simulink model "starshotsimv3p5"  (R2017a)
settings: Solver=ode45  StartTime=0.0  StopTime=30  MaxStep=4.0  MinStep=.001  RelTol=1e-6
values from neighbouring files (symbols this model uses):
  B0 = 3.12e-5    (= 3.12e-05)    [starshot_DC_KD_setup.m]    (also in starshot_DC_setup.m; starshotmath.m; temp.m)
  G = 6.67e-11    [starshot_DC_KD_setup.m]    (also in starshot_DC_setup.m; temp.m)
  M_Earth = 5.972e24    (= 5.972e+24)    [starshot_DC_KD_setup.m]    (also in starshot_DC_setup.m; temp.m)
  mu_0 = 4*pi*(10^-7)    (= 1.25663706144e-06)    [starshot_DC_KD_setup.m]    (also in starshot_DC_setup.m; temp.m)
  n = 1000    [starshot_DC_KD_setup.m]    (also in starshot_DC_setup.m; starshotmath.m; temp.m)
  q0 = [qmatlab(2:4),qmatlab(1)]'    [starshot_DC_KD_setup.m]    (also in starshot_DC_setup.m; temp.m)
  R_Earth = 6.378e6    (= 6378000)    [starshot_DC_KD_setup.m]    (also in starshot_DC_setup.m; temp.m)
undefined symbols (not defined in the file or in its folder): Kp_phi, omegacmd, quatcmd, starshot
libraries: vrlib x2
settings Model: Creator=armen  LastModifiedBy=armen

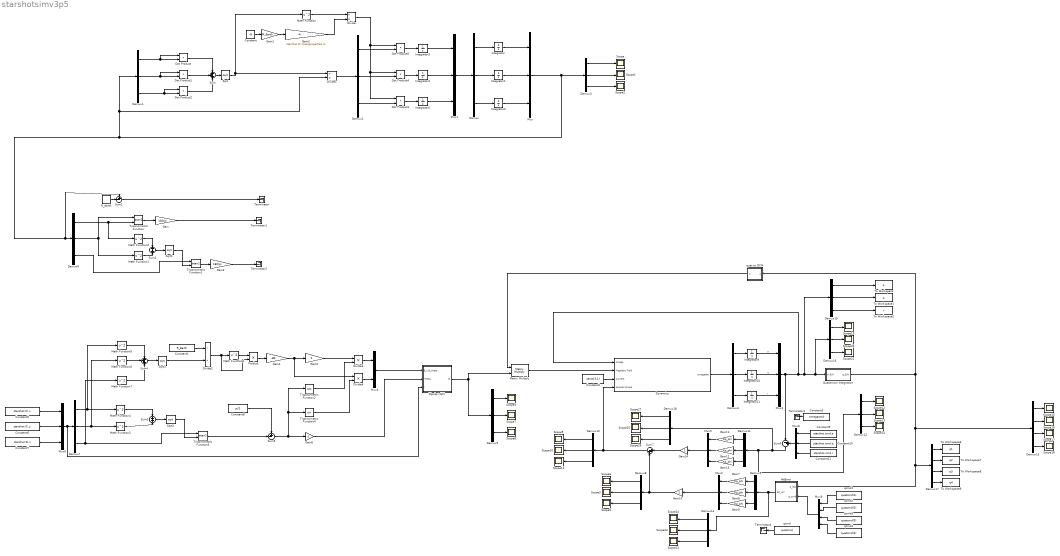
== system starshotsimv3p5 ==
  AttError : Subsystem
  Constant : Constant  Value=-G
  Constant1 : Constant  Value=R_Earth
  Constant10 : Constant  Value=starshot.cmd.q
  Constant11 : Constant  Value=starshot.cmd.r
  Constant2 : Constant  Value=zeros(3,1)
  Constant3 : Constant  Value=omegacmd
  Constant5 : Constant  Value=starshot.IC.x
  Constant6 : Constant  Value=starshot.IC.y
  Constant7 : Constant  Value=starshot.IC.z
  Constant8 : Constant  Value=pi/2
  Constant9 : Constant  Value=starshot.cmd.p
  Demux{,1..12,14..16,18} (17 alike) : Demux  Outputs=3
  Demux13 : Demux
  Demux17 : Demux
  Dipole->ECI : Subsystem
  Divide : Product  Inputs=/*
  Divide1 : Product  Inputs=/*
  Divide2 : Product  Inputs=*/
  Divide3 : Product  Inputs=**
  Divide4 : Product  Inputs=**
  Dot Product{,1..5} (6 alike) : DotProduct  InputSameDT=on  OutDataTypeStr=Inherit: Inherit via internal rule
  Dynamics : Subsystem
  Gain : Gain  Gain=180/pi
  Gain1 : Gain  Gain=M_Earth
  Gain10 : Gain
  Gain{7..9,11..13} (6 alike) : Gain  Gain=Kp_phi
  Gain14 : Gain
  Gain2 : Gain  Gain=starshot.IC.massproperties.m
  Gain3 : Gain  Gain=180/pi
  Gain4 : Gain  Gain=-B0
  Gain5 : Gain  Gain=2
  Gain6 : Gain  Gain=-1
  Integrator : Integrator  InitialCondition=starshot.IC.x
  Integrator1 : Integrator  InitialCondition=starshot.IC.y
  Integrator10 : Integrator  InitialCondition=starshot.IC.q
  Integrator11 : Integrator  InitialCondition=starshot.IC.r
  Integrator2 : Integrator  InitialCondition=starshot.IC.z
  Integrator3 : Integrator  InitialCondition=starshot.IC.xdot
  Integrator4 : Integrator  InitialCondition=starshot.IC.ydot
  Integrator5 : Integrator  InitialCondition=starshot.IC.zdot
  Integrator9 : Integrator  InitialCondition=starshot.IC.p
  Math Function{,1..8} (9 alike) : Math  Operator=square  SaturateOnIntegerOverflow=on
  Matrix Multiply : Product  Multiplication=Matrix(*)
  Mux{,1..3,5..6,8} (7 alike) : Mux  Inputs=3
  Mux4 : Mux  Inputs=2
  Mux9 : Mux
  Product : Product
  Quaternion Integration : Subsystem
  R_earth : Constant  Value=6.371e6
  Scope{,1..27} (28 alike) : Scope
  Sqrt{,1..3} (4 alike) : Sqrt  SaturateOnIntegerOverflow=on
  Sum : Sum  Inputs=+++
  Sum1 : Sum  Inputs=+-|
  Sum2 : Sum
  Sum3 : Sum
  Sum4 : Sum  Inputs=+++
  Sum5 : Sum  Inputs=+-|
  Sum6 : Sum  Inputs=|-+
  Sum7 : Sum  Inputs=|++
  Terminator{,1..4} (5 alike) : Terminator
  To Workspace : ToWorkspace  VariableName=p  SaveFormat=Timeseries  SampleTime=-1
  To Workspace1 : ToWorkspace  VariableName=q  SaveFormat=Timeseries  SampleTime=-1
  To Workspace2 : ToWorkspace  VariableName=r  SaveFormat=Timeseries  SampleTime=-1
  To Workspace6 : ToWorkspace  VariableName=q1  SaveFormat=Timeseries  SampleTime=-1
  To Workspace7 : ToWorkspace  VariableName=q2  SaveFormat=Timeseries  SampleTime=-1
  To Workspace8 : ToWorkspace  VariableName=q3  SaveFormat=Timeseries  SampleTime=-1
  To Workspace9 : ToWorkspace  VariableName=q4  SaveFormat=Timeseries  SampleTime=-1
  Trigonometric Function : Trigonometry  Operator=atan2
  Trigonometric Function1 : Trigonometry  Operator=atan2
  Trigonometric Function2 : Trigonometry  Operator=cos
  Trigonometric Function3 : Trigonometry  Operator=atan2
  Trigonometric Function4 : Trigonometry
  qcmd : Constant  Value=quatcmd
  qcmd1 : Constant  Value=quatcmd(1)
  qcmd2 : Constant  Value=quatcmd(2)
  qcmd3 : Constant  Value=quatcmd(3)
  qcmd4 : Constant  Value=quatcmd(4)
  quat to DCM : Subsystem  mask(Direction Cosine Matrix){}
      mask help: Determines the 3x3 Direction Cosine Matrix (DCM) from a 4x1 quaternion orientation vector. The outputted DCM transforms vectors from inertial axes to body axes. This version corrects the fucked-up MATLAB one.
      mask Help:
      | <p>This block determines the 3x3 Direction Cosine Matrix (DCM) from a 4x1 quaternion orientation vector. The outputted DCM transforms vectors from inertial axes to body axes.  This version corrects the fucked-up MATLAB one</p>
      | 
      | <p>The block input and output contain more than one signal as described below.</p>
      | 
      | <p><H4>Block Vector Input - Quaternion</H4>
      | <ul>
      | <li>q0</li>
      | <li>q1</li>
      | <li>q2</li>
      | <li>q3</li>
      | </ul>
      | </p>
      | 
      | <p><H4>Block Matrix Output - Direction Cosine Matrix  </H4>
      |     <ul>
      |    </ul>
      |    </p>
      mask Display: disp('q to Q')
  wires:
  Integrator/1 -> Mux/1
  Integrator2/1 -> Mux/3
  Integrator1/1 -> Mux/2
  Demux/3 -> Integrator2/1
  Demux/2 -> Integrator1/1
  Demux/1 -> Integrator/1
  Mux1/1 -> Demux/1
  Integrator5/1 -> Mux1/3
  Integrator4/1 -> Mux1/2
  Integrator3/1 -> Mux1/1
  Demux1/1 -> Dot Product/1, Dot Product/2
  Demux1/2 -> Dot Product1/1, Dot Product1/2
  Demux1/3 -> Dot Product2/1, Dot Product2/2
  Dot Product1/1 -> Sum/2
  Dot Product2/1 -> Sum/3
  Dot Product/1 -> Sum/1
  Sum/1 -> Sqrt/1
  Constant/1 -> Gain1/1
  Sqrt/1 -> Math Function/1, Divide1/1
  Gain1/1 -> Gain2/1
  Gain2/1 -> Divide/2
  Math Function/1 -> Divide/1
  Divide/1 -> Dot Product3/1, Dot Product4/1, Dot Product5/1
  Demux2/3 -> Dot Product3/2
  Demux2/2 -> Dot Product4/2
  Demux2/1 -> Dot Product5/2
  Dot Product5/1 -> Integrator3/1
  Dot Product4/1 -> Integrator4/1
  Dot Product3/1 -> Integrator5/1
  Divide1/1 -> Demux2/1
  Demux3/1 -> Scope/1
  Demux3/2 -> Scope1/1
  Demux3/3 -> Scope2/1
  Integrator9/1 -> Mux3/1  "p"
  Integrator10/1 -> Mux3/2  "q"
  Integrator11/1 -> Mux3/3  "r"
  Demux4/3 -> Integrator11/1
  Demux4/2 -> Integrator10/1
  Demux4/1 -> Integrator9/1
  Sum1/1 -> Terminator/1
  R_earth/1 -> Sum1/2
  Demux6/1 -> Math Function2/1, Trigonometric Function/2
  Demux6/2 -> Trigonometric Function/1, Math Function1/1
  Demux6/3 -> Trigonometric Function1/1
  Math Function2/1 -> Sum2/1
  Math Function1/1 -> Sum2/2
  Sum2/1 -> Sqrt1/1
  Sqrt1/1 -> Trigonometric Function1/2
  Trigonometric Function/1 -> Gain/1
  Trigonometric Function1/1 -> Gain3/1
  Gain/1 -> Terminator1/1
  Gain3/1 -> Terminator2/1
  Dynamics/1(omegadot) -> Demux4/1
  Sqrt2/1 -> Trigonometric Function3/2
  Sum3/1 -> Sqrt2/1
  Math Function3/1 -> Sum3/2
  Math Function4/1 -> Sum3/1
  Demux7/3 -> Math Function7/1, Trigonometric Function3/1
  Demux7/2 -> Math Function6/1, Math Function3/1
  Demux7/1 -> Math Function5/1, Math Function4/1
  Mux/1 -> Sum1/1, Demux6/1, Divide1/2, Demux1/1, Demux3/1
  Math Function6/1 -> Sum4/2
  Math Function5/1 -> Sum4/1
  Math Function7/1 -> Sum4/3
  Sum4/1 -> Sqrt3/1
  Sqrt3/1 -> Divide2/2
  Constant1/1 -> Divide2/1
  Divide2/1 -> Product/2, Math Function8/1
  Math Function8/1 -> Product/1
  Product/1 -> Gain4/1
  Gain4/1 -> Gain5/1, Divide4/1
  Gain5/1 -> Divide3/1
  Trigonometric Function2/1 -> Divide3/2
  Trigonometric Function4/1 -> Divide4/2
  Divide3/1 -> Mux4/1
  Divide4/1 -> Mux4/2
  Mux4/1 -> Dipole->ECI/1(B_r,B_theta)
  Gain6/1 -> Dipole->ECI/2(-theta)
  Demux9/3 -> Scope8/1
  Demux9/1 -> Scope4/1
  Demux9/2 -> Scope7/1
  Dipole->ECI/1(B) -> Matrix Multiply/2, Demux9/1
  Mux6/1 -> Dipole->ECI/3(r), Demux7/1
  Constant7/1 -> Mux6/3
  Constant6/1 -> Mux6/2
  Constant5/1 -> Mux6/1
  Trigonometric Function3/1 -> Sum5/2
  Constant8/1 -> Sum5/1
  Sum5/1 -> Trigonometric Function2/1, Trigonometric Function4/1, Gain6/1
  AttError/1(att_err) -> Demux14/1, Demux5/1
  Mux2/1 -> Gain10/1
  qcmd/1 -> Terminator4/1
  Gain7/1 -> Mux2/1
  Demux5/1 -> Gain7/1
  Gain8/1 -> Mux2/2
  Demux5/2 -> Gain8/1
  Gain9/1 -> Mux2/3
  Demux5/3 -> Gain9/1
  Constant2/1 -> Dynamics/3("Current ")
  Demux10/1 -> Scope9/1
  Demux10/2 -> Scope10/1
  Demux10/3 -> Scope11/1
  Demux11/3 -> Gain13/1
  Gain13/1 -> Mux5/3
  Demux11/2 -> Gain12/1
  Gain12/1 -> Mux5/2
  Demux11/1 -> Gain11/1
  Gain11/1 -> Mux5/1
  Mux5/1 -> Gain14/1
  Constant3/1 -> Terminator3/1
  Gain14/1 -> Sum7/1
  Sum7/1 -> Dynamics/4(pseudo-torque), Demux10/1
  Demux12/3 -> Scope14/1
  Demux12/1 -> Scope12/1
  Demux12/2 -> Scope13/1
  Demux13/1 -> Scope15/1
  Demux13/4 -> Scope18/1
  Demux13/3 -> Scope17/1
  Quaternion Integration/1(q_B/N) -> Demux13/1, AttError/1(q_est), Demux17/1, quat to DCM/1(e0 e1 e2 e3)
  Demux13/2 -> Scope16/1
  Demux15/3 -> To Workspace2/1
  Demux15/2 -> To Workspace1/1
  Demux15/1 -> To Workspace/1
  Sum6/1 -> Demux18/1, Demux12/1, Demux11/1
  Demux17/3 -> To Workspace8/1
  Demux17/2 -> To Workspace7/1
  Demux17/1 -> To Workspace6/1
  Demux17/4 -> To Workspace9/1
  Mux8/1 -> Sum6/2
  Constant10/1 -> Mux8/2
  Constant11/1 -> Mux8/3
  Constant9/1 -> Mux8/1
  Mux9/1 -> AttError/2(q_cmd)
  qcmd1/1 -> Mux9/1
  qcmd2/1 -> Mux9/2
  qcmd3/1 -> Mux9/3
  qcmd4/1 -> Mux9/4
  Mux3/1 -> Demux16/1, Quaternion Integration/1(w B/N), Demux15/1, Dynamics/1(omega), Sum6/1
  Demux16/2 -> Scope20/1
  Demux16/1 -> Scope19/1
  Demux16/3 -> Scope21/1
  quat to DCM/1(DCM) -> Matrix Multiply/1
  Matrix Multiply/1 -> Dynamics/2(Magnetic Field)
  Gain10/1 -> Demux8/1, Sum7/2
  Demux8/3 -> Scope5/1
  Demux8/2 -> Scope3/1
  Demux8/1 -> Scope6/1
  Demux14/1 -> Scope24/1
  Demux14/2 -> Scope22/1
  Demux14/3 -> Scope23/1
  Demux18/3 -> Scope26/1
  Demux18/2 -> Scope25/1
  Demux18/1 -> Scope27/1

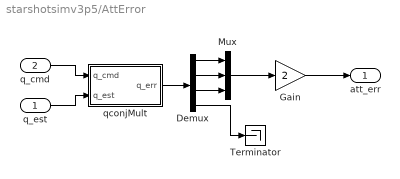
== system starshotsimv3p5/AttError ==
  q_est : Inport  PortDimensions=4
  q_cmd : Inport  Port=2  PortDimensions=4
  Demux : Demux
  Gain : Gain  Gain=2  SaturateOnIntegerOverflow=on  OutDataTypeStr=Inherit: Same as input  ParamDataTypeStr=Inherit: Same as input
  Mux : Mux  Inputs=3
  Terminator : Terminator
  qconjMult : Subsystem
  att_err : Outport
  wires:
  Demux/4 -> Terminator/1
  Gain/1 -> att_err/1
  Mux/1 -> Gain/1
  Demux/3 -> Mux/3
  Demux/2 -> Mux/2
  Demux/1 -> Mux/1
  qconjMult/1(q_err) -> Demux/1
  q_est/1 -> qconjMult/2(q_est)
  q_cmd/1 -> qconjMult/1(q_cmd)

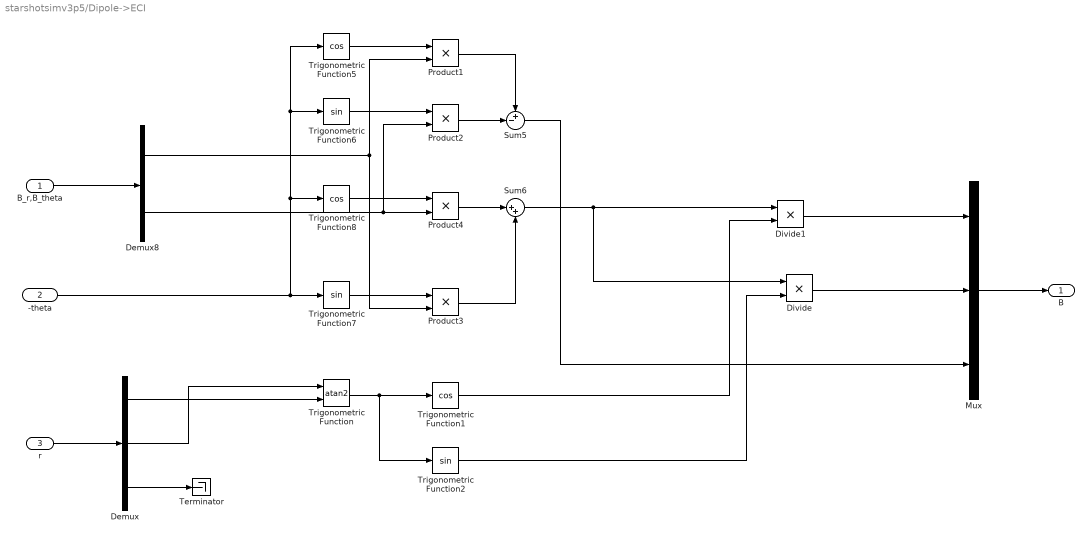
== system starshotsimv3p5/Dipole->ECI ==
  B_r,B_theta : Inport
  -theta : Inport  Port=2
  r : Inport  Port=3
  Demux : Demux  Outputs=3
  Demux8 : Demux  Outputs=2
  Divide : Product  Inputs=**
  Divide1 : Product  Inputs=**
  Mux : Mux  Inputs=3
  Product{1..4} (4 alike) : Product
  Sum5 : Sum  Inputs=+-|
  Sum6 : Sum  Inputs=|++
  Terminator : Terminator
  Trigonometric Function : Trigonometry  Operator=atan2
  Trigonometric Function1 : Trigonometry  Operator=cos
  Trigonometric Function2 : Trigonometry
  Trigonometric Function5 : Trigonometry  Operator=cos
  Trigonometric Function6 : Trigonometry
  Trigonometric Function7 : Trigonometry
  Trigonometric Function8 : Trigonometry  Operator=cos
  B : Outport
  wires:
  -theta/1 -> Trigonometric Function5/1, Trigonometric Function6/1, Trigonometric Function8/1, Trigonometric Function7/1
  Product4/1 -> Sum6/1
  Product3/1 -> Sum6/2
  Demux8/1 -> Product3/2, Product1/2
  Demux8/2 -> Product2/2, Product4/2
  Trigonometric Function5/1 -> Product1/1
  Product2/1 -> Sum5/2
  Trigonometric Function7/1 -> Product3/1
  B_r,B_theta/1 -> Demux8/1
  Sum5/1 -> Mux/3
  Trigonometric Function8/1 -> Product4/1
  Trigonometric Function6/1 -> Product2/1
  Sum6/1 -> Divide1/1, Divide/1
  Product1/1 -> Sum5/1
  r/1 -> Demux/1
  Demux/3 -> Terminator/1
  Demux/2 -> Trigonometric Function/1
  Demux/1 -> Trigonometric Function/2
  Trigonometric Function/1 -> Trigonometric Function1/1, Trigonometric Function2/1
  Trigonometric Function1/1 -> Divide1/2
  Trigonometric Function2/1 -> Divide/2
  Mux/1 -> B/1
  Divide1/1 -> Mux/1
  Divide/1 -> Mux/2

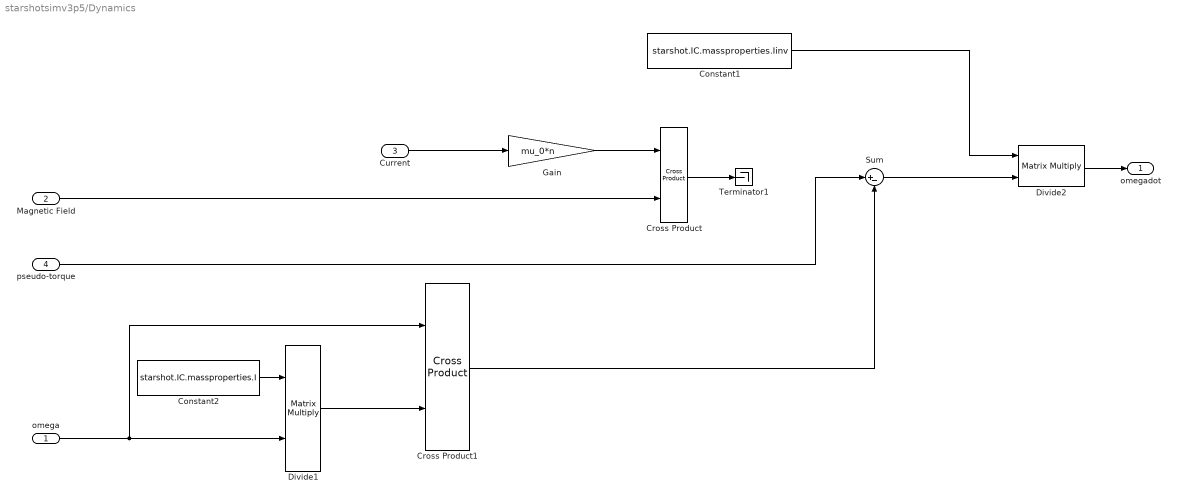
== system starshotsimv3p5/Dynamics ==
  omega : Inport
  Magnetic Field : Inport  Port=2
  "Current " : Inport  Port=3
  pseudo-torque : Inport  Port=4
  Constant1 : Constant  Value=starshot.IC.massproperties.Iinv  VectorParams1D=off
  Constant2 : Constant  Value=starshot.IC.massproperties.I  VectorParams1D=off
  Cross Product : vrlib/Utilities/Cross Product
      settings: SourceProductBaseCode=VR
  Cross Product1 : vrlib/Utilities/Cross Product
      settings: SourceProductBaseCode=VR
  Divide1 : Product  Inputs=**  Multiplication=Matrix(*)
  Divide2 : Product  Inputs=**  Multiplication=Matrix(*)
  Gain : Gain  Gain=mu_0*n
  Sum : Sum  Inputs=|+-
  Terminator1 : Terminator
  omegadot : Outport
  wires:
  omega/1 -> Divide1/2, Cross Product1/1
  Constant2/1 -> Divide1/1
  "Current "/1 -> Gain/1
  Magnetic Field/1 -> Cross Product/2
  Gain/1 -> Cross Product/1
  Cross Product/1 -> Terminator1/1
  Divide1/1 -> Cross Product1/2
  Cross Product1/1 -> Sum/2
  Sum/1 -> Divide2/2
  Constant1/1 -> Divide2/1
  Divide2/1 -> omegadot/1
  pseudo-torque/1 -> Sum/1

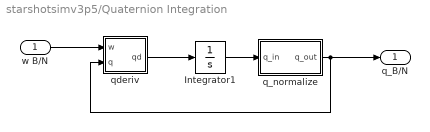
== system starshotsimv3p5/Quaternion Integration ==
  w B/N : Inport
  Integrator1 : Integrator  InitialCondition=q0
  q_normalize : Subsystem
  qderiv : Subsystem
  q_B/N : Outport
  wires:
  w B/N/1 -> qderiv/1(w)
  q_normalize/1(q_out) -> qderiv/2(q), q_B/N/1
  Integrator1/1 -> q_normalize/1(q_in)
  qderiv/1(qd) -> Integrator1/1

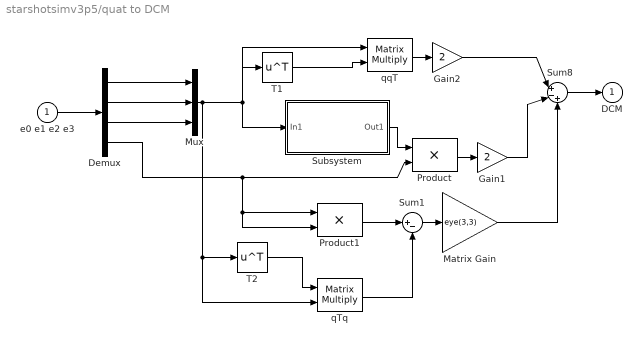
== system starshotsimv3p5/quat to DCM ==
  e0 e1 e2 e3 : Inport
  Demux : Demux
  Gain1 : Gain  Gain=2  SaturateOnIntegerOverflow=on  OutDataTypeStr=Inherit: Same as input  ParamDataTypeStr=Inherit: Same as input
  Gain2 : Gain  Gain=2  SaturateOnIntegerOverflow=on  OutDataTypeStr=Inherit: Same as input  ParamDataTypeStr=Inherit: Same as input
  Matrix Gain : Gain  Gain=eye(3,3)  SaturateOnIntegerOverflow=on  OutDataTypeStr=Inherit: Same as input  ParamDataTypeStr=Inherit: Same as input
  Mux : Mux  Inputs=3
  Product : Product  SaturateOnIntegerOverflow=on  InputSameDT=on  OutDataTypeStr=Inherit: Same as first input
  Product1 : Product  SaturateOnIntegerOverflow=on  InputSameDT=on  OutDataTypeStr=Inherit: Same as first input
  Subsystem : Subsystem
      mask Display: disp('3x3 cross matrix')
  Sum1 : Sum  Inputs=|+-  SaturateOnIntegerOverflow=on  InputSameDT=on  OutDataTypeStr=Inherit: Same as first input
  Sum8 : Sum  Inputs=|+-+  SaturateOnIntegerOverflow=on  InputSameDT=on  OutDataTypeStr=Inherit: Same as first input
  T1 : Math  Operator=transpose  SaturateOnIntegerOverflow=on
  T2 : Math  Operator=transpose  SaturateOnIntegerOverflow=on
  qTq : Product  Multiplication=Matrix(*)  SaturateOnIntegerOverflow=on  InputSameDT=on  OutDataTypeStr=Inherit: Same as first input
  qqT : Product  Multiplication=Matrix(*)  SaturateOnIntegerOverflow=on  InputSameDT=on  OutDataTypeStr=Inherit: Same as first input
  DCM : Outport  InitialOutput=0
  wires:
  Subsystem/1(Out1) -> Product/1
  Matrix Gain/1 -> Sum8/3
  Sum1/1 -> Matrix Gain/1
  qTq/1 -> Sum1/2
  T2/1 -> qTq/1
  Product1/1 -> Sum1/1
  Gain1/1 -> Sum8/2
  Gain2/1 -> Sum8/1
  qqT/1 -> Gain2/1
  T1/1 -> qqT/2
  Product/1 -> Gain1/1
  Mux/1 -> qTq/2, T2/1, Subsystem/1(In1), qqT/1, T1/1
  Demux/4 -> Product1/2, Product1/1, Product/2
  Demux/3 -> Mux/3
  Demux/2 -> Mux/2
  Demux/1 -> Mux/1
  e0 e1 e2 e3/1 -> Demux/1
  Sum8/1 -> DCM/1

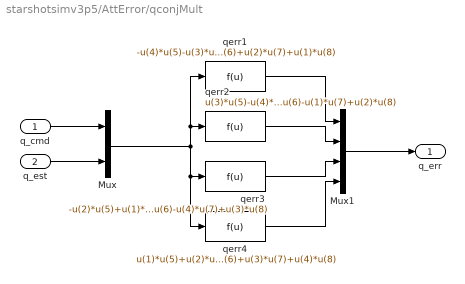
== system starshotsimv3p5/AttError/qconjMult ==
  q_cmd : Inport
  q_est : Inport  Port=2
  Mux : Mux  Inputs=2
  Mux1 : Mux
  qerr1 : Fcn  Expr=-u(4)*u(5)-u(3)*u(6)+u(2)*u(7)+u(1)*u(8)
  qerr2 : Fcn  Expr=u(3)*u(5)-u(4)*u(6)-u(1)*u(7)+u(2)*u(8)
  qerr3 : Fcn  Expr=-u(2)*u(5)+u(1)*u(6)-u(4)*u(7)+u(3)*u(8)
  qerr4 : Fcn  Expr=u(1)*u(5)+u(2)*u(6)+u(3)*u(7)+u(4)*u(8)
  q_err : Outport
  wires:
  Mux1/1 -> q_err/1
  qerr4/1 -> Mux1/4
  qerr3/1 -> Mux1/3
  qerr2/1 -> Mux1/2
  qerr1/1 -> Mux1/1
  Mux/1 -> qerr4/1, qerr3/1, qerr2/1, qerr1/1
  q_est/1 -> Mux/2
  q_cmd/1 -> Mux/1

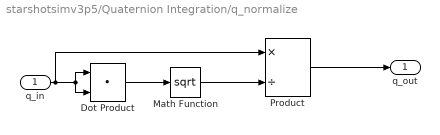
== system starshotsimv3p5/Quaternion Integration/q_normalize ==
  q_in : Inport  PortDimensions=4
  Dot Product : DotProduct  InputSameDT=on  OutDataTypeStr=Inherit: Inherit via internal rule
  Math Function : Math  Operator=sqrt  SaturateOnIntegerOverflow=on
  Product : Product  Inputs=*/  SaturateOnIntegerOverflow=on  InputSameDT=on  OutDataTypeStr=Inherit: Same as first input
  q_out : Outport
  wires:
  Product/1 -> q_out/1
  Math Function/1 -> Product/2
  Dot Product/1 -> Math Function/1
  q_in/1 -> Dot Product/2, Dot Product/1, Product/1

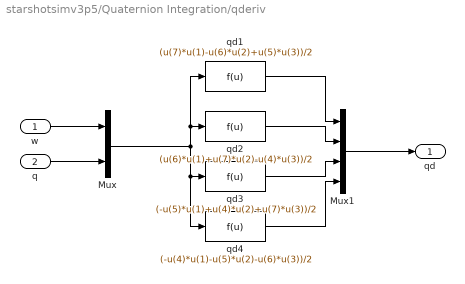
== system starshotsimv3p5/Quaternion Integration/qderiv ==
  w : Inport
  q : Inport  Port=2
  Mux : Mux  Inputs=2
  Mux1 : Mux
  qd1 : Fcn  Expr=(u(7)*u(1)-u(6)*u(2)+u(5)*u(3))/2
  qd2 : Fcn  Expr=(u(6)*u(1)+u(7)*u(2)-u(4)*u(3))/2
  qd3 : Fcn  Expr=(-u(5)*u(1)+u(4)*u(2)+u(7)*u(3))/2
  qd4 : Fcn  Expr=(-u(4)*u(1)-u(5)*u(2)-u(6)*u(3))/2
  qd : Outport
  wires:
  Mux1/1 -> qd/1
  qd4/1 -> Mux1/4
  qd3/1 -> Mux1/3
  qd2/1 -> Mux1/2
  qd1/1 -> Mux1/1
  Mux/1 -> qd4/1, qd3/1, qd2/1, qd1/1
  q/1 -> Mux/2
  w/1 -> Mux/1

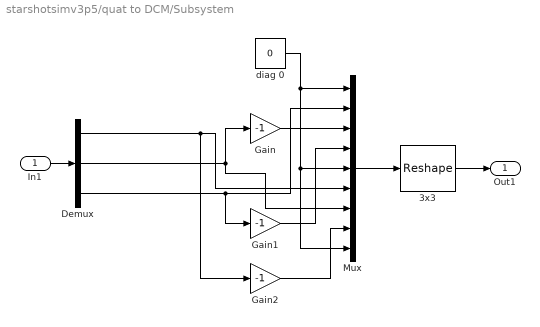
== system starshotsimv3p5/quat to DCM/Subsystem ==
  In1 : Inport
  3x3 : Reshape  OutputDimensionality=Customize  OutputDimensions=[3,3]
  Demux : Demux  Outputs=3
  Gain : Gain  Gain=-1  SaturateOnIntegerOverflow=on  OutDataTypeStr=Inherit: Same as input  ParamDataTypeStr=Inherit: Same as input
  Gain1 : Gain  Gain=-1  SaturateOnIntegerOverflow=on  OutDataTypeStr=Inherit: Same as input  ParamDataTypeStr=Inherit: Same as input
  Gain2 : Gain  Gain=-1  SaturateOnIntegerOverflow=on  OutDataTypeStr=Inherit: Same as input  ParamDataTypeStr=Inherit: Same as input
  Mux : Mux  Inputs=9
  "diag 0 " : Constant  Value=0
  Out1 : Outport
  wires:
  Gain2/1 -> Mux/8
  Demux/1 -> Gain2/1, Mux/6
  Gain1/1 -> Mux/4
  Demux/2 -> Mux/7, Gain/1
  Gain/1 -> Mux/3
  Demux/3 -> Gain1/1, Mux/2
  Mux/1 -> 3x3/1
  "diag 0 "/1 -> Mux/9, Mux/5, Mux/1
  3x3/1 -> Out1/1
  In1/1 -> Demux/1
